simulink model "DelayLine"  (R2020b)
settings: Solver=ode45  StartTime=0.0  StopTime=3  FixedStep=0.0002  RelTol=1e-6
undefined symbols (not defined in the file or in its folder): S
libraries: simrfV2util1 x32, simrfV2elements x32, simrfV2_lib x1
settings Model: Creator=tian  LastModifiedBy=tian
settings SolverCC: ZeroCrossAlgorithm=Adaptive
settings DebuggingCC: IgnoredZcDiagnostic=none

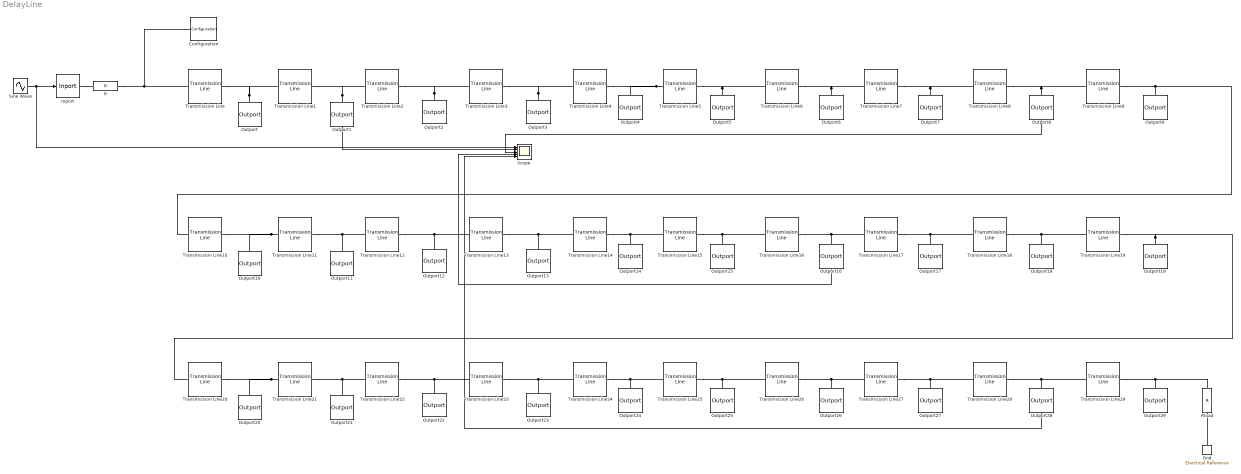
== system DelayLine ==
  Configuration : simrfV2util1/Configuration  AutoFreq=on  Tones=[0] Hz  Harmonics=[1]  NormalizeCarrierPower=on  SolverType=Auto  UseCCode=on  StepSize=10e-6 s  AddNoise=on  defaultRNG=on  Seed=0  Temperature=290 K  SolverDelFlag=0  AbsTol=1e-6  RelTol=1e-3  MaxIter=10  ErrorEstimationType=2-norm over all variables  EnableInterpFilter=on  HiddenFIRfilterControllerParam=on  SmallSignalApprox=off  AllSimFreqs=on  SimFreqs=[] Hz  SimFreqsInternal=[]  SamplesPerFrame=1
      settings: SourceProductBaseCode=RB
  Gnd : simrfV2_lib/Elements/Electrical Reference
      settings: SourceProductBaseCode=RB  InternalSimscapePortConfiguration="{\"Bottom\":[],\"Left\":[{\"id\":\"V\",\"label\":\"\",\"type\":\"foundation.rf.circuitenvelope\"}],\"Right\":[],\"Top\":[]}"
  Inport : simrfV2util1/Inport  SimulinkInputSignalType=Ideal voltage  CarrierFreq=0 Hz  ZS=0  InternalGrounding=on
      settings: SourceProductBaseCode=RB
  Outport{,1..29} (30 alike) : simrfV2util1/Outport  SensorType=Ideal voltage  OutputFormat=Real Passband  CarrierFreq=0 Hz  ZL=Inf  InternalGrounding=on  StepSize=1e-06 s  AutoStep=on
      settings: SourceProductBaseCode=RB
  R : simrfV2elements/R  classname=resistor  Resistance=135 Ohm  AddNoise=on
      settings: SourceProductBaseCode=RB
  Rload : simrfV2elements/R  classname=resistor  Resistance=135 Ohm  AddNoise=on
      settings: SourceProductBaseCode=RB
  Scope : Scope  NumInputPorts=5
  Sine Wave : Sin  Frequency=20  SampleTime=0
  Transmission Line{,1..29} (30 alike) : simrfV2elements/Transmission Line  classname=xline  Model_type=Delay-based and lossy  Parameterization=By inductance and capacitance  TransDelay=0.06 s  CharImped=135 Ohm  Resistance=10 Ohm/m  Inductance=235e-9 H/m  Capacitance=94e-12 F/m  Conductance=5e-6 S/m  LineLength=1 m  NumSegments=1  InternalGrounding=on  OuterRadius=2.57 mm  InnerRadius=0.725 mm  MuR=1  EpsilonR=2.2  LossTangent=0  SigmaCond=inf S/m  StubMode=Not a stub  Termination=Open  ConductorWidth=0.6 mm  SlotWidth=0.2 mm  Height=0.635 mm  Thickness=5 um  SWidth=0.6 mm  Radius=0.67 mm  Separation=1.62 mm  PWidth=5 mm  PSeparation=1 mm  PV=299792458  Loss=1  SourceFreq=User-specified  PlotFreq=[1e9:1e6:3e9] Hz  PlotType=X-Y plane  YParam1=S(1,1)  YFormat1=Magnitude (decibels)  YParam2=S(2,2)  YFormat2=Magnitude (decibels)  YOption=Linear  XOption=Linear  FitOpt=Share all poles  FitTol=-40  SparamRepresentation=Frequency domain  Freq=1e9 Hz  Interp_type=Linear  AutoImpulseLength=off  ImpulseLength=0 s  MagModeling=off
      settings: SourceProductBaseCode=RB
  wires:
  Sine Wave/1 -> Scope/1, Inport/1
  Outport1/1 -> Scope/2
  Outport8/1 -> Scope/3
  Outport16/1 -> Scope/4
  Outport28/1 -> Scope/5
  connections:
  Inport/RConn1 -- R/LConn1
  Transmission Line11/LConn1 -- Outport10/LConn1 -- Transmission Line10/RConn1
  Outport/LConn1 -- Transmission Line/RConn1 -- Transmission Line1/LConn1
  Transmission Line16/LConn1 -- Outport15/LConn1 -- Transmission Line15/RConn1
  Outport7/LConn1 -- Transmission Line7/RConn1 -- Transmission Line8/LConn1
  Transmission Line29/LConn1 -- Outport28/LConn1 -- Transmission Line28/RConn1
  Transmission Line23/LConn1 -- Outport22/LConn1 -- Transmission Line22/RConn1
  Transmission Line27/LConn1 -- Outport26/LConn1 -- Transmission Line26/RConn1
  Transmission Line14/RConn1 -- Transmission Line15/LConn1 -- Outport14/LConn1
  Transmission Line23/RConn1 -- Outport23/LConn1 -- Transmission Line24/LConn1
  Transmission Line29/RConn1 -- Rload/LConn1 -- Outport29/LConn1
  Transmission Line28/LConn1 -- Outport27/LConn1 -- Transmission Line27/RConn1
  Transmission Line12/LConn1 -- Outport11/LConn1 -- Transmission Line11/RConn1
  Transmission Line13/LConn1 -- Outport12/LConn1 -- Transmission Line12/RConn1
  Outport8/LConn1 -- Transmission Line8/RConn1 -- Transmission Line9/LConn1
  Transmission Line22/LConn1 -- Outport21/LConn1 -- Transmission Line21/RConn1
  Transmission Line24/RConn1 -- Transmission Line25/LConn1 -- Outport24/LConn1
  Outport5/LConn1 -- Transmission Line5/RConn1 -- Transmission Line6/LConn1
  Transmission Line18/LConn1 -- Outport17/LConn1 -- Transmission Line17/RConn1
  Outport19/LConn1 -- Transmission Line19/RConn1 -- Transmission Line20/LConn1
  Transmission Line17/LConn1 -- Outport16/LConn1 -- Transmission Line16/RConn1
  Outport6/LConn1 -- Transmission Line6/RConn1 -- Transmission Line7/LConn1
  Outport2/LConn1 -- Transmission Line2/RConn1 -- Transmission Line3/LConn1
  Transmission Line13/RConn1 -- Outport13/LConn1 -- Transmission Line14/LConn1
  Outport3/LConn1 -- Transmission Line3/RConn1 -- Transmission Line4/LConn1
  Outport1/LConn1 -- Transmission Line1/RConn1 -- Transmission Line2/LConn1
  Transmission Line19/LConn1 -- Outport18/LConn1 -- Transmission Line18/RConn1
  Transmission Line26/LConn1 -- Outport25/LConn1 -- Transmission Line25/RConn1
  Transmission Line21/LConn1 -- Outport20/LConn1 -- Transmission Line20/RConn1
  Transmission Line5/LConn1 -- Transmission Line4/RConn1 -- Outport4/LConn1
  Transmission Line10/LConn1 -- Transmission Line9/RConn1 -- Outport9/LConn1
  R/RConn1 -- Configuration/LConn1 -- Transmission Line/LConn1
  Gnd/LConn1 -- Rload/RConn1
